simulink model "Energy"  (R2024b)
settings: Solver=ode1  StartTime=0.0  StopTime=955800  FixedStep=1  RelTol=1e-3
(part 3 of 3)

== matlab function Energy/Subsystem2/DCDC1_2 ==
  data: V_out input; I_in input; V_in input; I_out output
function I_out = fcn(V_out,I_in, V_in)
%% DCDC模型 - 输入电流计算输出电流
%% 输入:
%%   I_in  - 输入电流 (A)
%%   V_in  - 输入电压 (V)
%%   V_out - 输出电压 (V)
%% 输出:
%%   I_out - 输出电流 (A)

%% ===== 效率MAP表 =====
% 输入电压断点 (V)
V_bp = [160, 180, 200, 220, 240, 260, 280];

% 输入电流断点 (A)
I_bp = [0, 20, 40, 60, 80, 100, 120, 140, 160, 180, 200];

% 效率表 (%)，行=电流，列=电压
Eta_map = [
    86, 86, 86, 86, 86, 86, 86;
    88, 88, 87, 87, 87, 87, 86;
    92, 91, 91, 90, 89, 88, 87;
    94, 93, 93, 92, 91, 90, 88;
    94.5, 94, 94, 93, 92, 91, 89;
    95, 94.5, 94, 93.5, 93, 91, 90;
    95, 94.5, 94.5, 94, 93, 92, 91;
    95, 95, 94.5, 94, 93.5, 93, 91;
    95, 95, 94.5, 94, 93, 92, 91;
    95, 94.5, 94.5, 93, 92, 91, 91;
    95, 94.5, 94, 92, 91, 91, 91
] / 100;

%% ===== 输入限幅 =====
V_in_clamp = max(160, min(280, V_in));
I_in_clamp = max(0, min(200, I_in));

%% ===== 查表获取效率 =====
% 找电压区间
nV = 7;
jV = 1;
for j = 1:nV-1
    if V_in_clamp >= V_bp(j) && V_in_clamp <= V_bp(j+1)
        jV = j;
        break;
    end
end
if V_in_clamp >= V_bp(nV)
    jV = nV - 1;
end
tV = (V_in_clamp - V_bp(jV)) / (V_bp(jV+1) - V_bp(jV));

% 找电流区间
nI = 11;
iI = 1;
for i = 1:nI-1
    if I_in_clamp >= I_bp(i) && I_in_clamp <= I_bp(i+1)
        iI = i;
        break;
    end
end
if I_in_clamp >= I_bp(nI)
    iI = nI - 1;
end
tI = (I_in_clamp - I_bp(iI)) / (I_bp(iI+1) - I_bp(iI));

% 双线性插值
eta_11 = Eta_map(iI, jV);
eta_12 = Eta_map(iI, jV+1);
eta_21 = Eta_map(iI+1, jV);
eta_22 = Eta_map(iI+1, jV+1);

eta_1 = eta_11 + tV * (eta_12 - eta_11);
eta_2 = eta_21 + tV * (eta_22 - eta_21);
eta = eta_1 + tI * (eta_2 - eta_1);

%% ===== 计算输出电流 =====
P_in = V_in * I_in;
P_out = P_in * eta;
V_out_safe = max(V_out, 1);
I_out = P_out / V_out_safe;

end
